simulink model "Rocket_Active_Airbrake_6DOF"  (R2026a)
settings: Solver=ode4  StopTime=28.0  FixedStep=0.002
PreLoadFcn:
  | init_airbrake_params
settings Model: Creator=wen-chungcheng  LastModifiedBy=wen-chungcheng

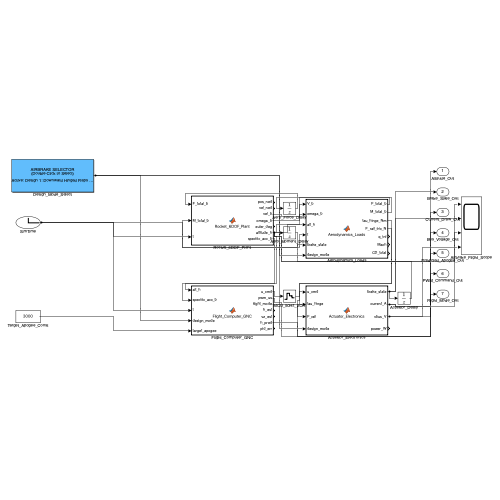
[thumbnail: Simulink's stored preview of the top-level diagram]
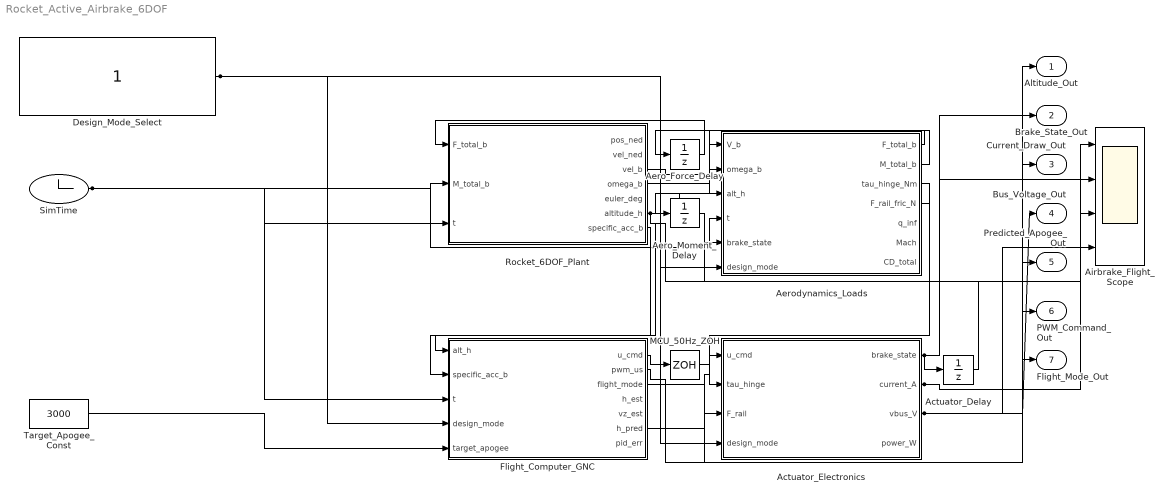
== system Rocket_Active_Airbrake_6DOF ==
  Actuator_Delay : UnitDelay  SampleTime=0.002
  Actuator_Electronics : MATLAB Function  TreatAsAtomicUnit=on
  Aero_Force_Delay : UnitDelay  InitialCondition=[0; 0; 0]  SampleTime=0.002
  Aero_Moment_Delay : UnitDelay  InitialCondition=[0; 0; 0]  SampleTime=0.002
  Aerodynamics_Loads : MATLAB Function  TreatAsAtomicUnit=on
  Airbrake_Flight_Scope : Scope  NumInputPorts=4
  Design_Mode_Select : Constant  mask(Airbrake Design Selector){design_popup=Design 1: Downward Hinged Flaps (0 - 90 deg, Savox SC-1258TG)}
      mask prompts: design_popup "Active Airbrake Mechanism:"
      mask help:
      | Choose active airbrake mechanism for 6-DOF simulation:
      | - Design 1: Downward Hinged Flaps (0 to 90 deg, Savox SC-1258TG)
      | - Design 2: Radially Outward Sliding Flaps (90 deg constant, Actuonix L16-R)
      mask init:
      | choice = get_param(gcb, 'design_popup');
      | if contains(choice, 'Design 1')
      |     val_internal = 1;
      | else
      |     val_internal = 2;
      | end
      settings: OpenFcn=open_system(gcb, 'mask');
      mask TypeOptions design_popup: Design 1: Downward Hinged Flaps (0 - 90 deg, Savox SC-1258TG) | Design 2: Radially Outward Sliding Flaps (90 deg, Actuonix L16-R)
      mask Display: disp(sprintf('AIRBRAKE SELECTOR\\n(Double-Click to Select)\\n\\nActive: %s', design_popup));
  Flight_Computer_GNC : MATLAB Function  TreatAsAtomicUnit=on
  MCU_50Hz_ZOH : ZeroOrderHold  SampleTime=0.02
  Rocket_6DOF_Plant : MATLAB Function  TreatAsAtomicUnit=on
  SimTime : Clock
  Target_Apogee_Const : Constant  Value=3000
  Altitude_Out : Outport
  Brake_State_Out : Outport  Port=2
  Current_Draw_Out : Outport  Port=3
  Bus_Voltage_Out : Outport  Port=4
  Predicted_Apogee_Out : Outport  Port=5
  PWM_Command_Out : Outport  Port=6
  Flight_Mode_Out : Outport  Port=7
  wires:
  SimTime/1 -> Rocket_6DOF_Plant/3(t), Aerodynamics_Loads/4(t), Flight_Computer_GNC/3(t)
  Design_Mode_Select/1 -> Aerodynamics_Loads/6(design_mode), Actuator_Electronics/4(design_mode), Flight_Computer_GNC/4(design_mode)
  Target_Apogee_Const/1 -> Flight_Computer_GNC/5(target_apogee)
  Aerodynamics_Loads/1(F_total_b) -> Aero_Force_Delay/1
  Aero_Force_Delay/1 -> Rocket_6DOF_Plant/1(F_total_b)
  Aerodynamics_Loads/2(M_total_b) -> Aero_Moment_Delay/1
  Aero_Moment_Delay/1 -> Rocket_6DOF_Plant/2(M_total_b)
  Rocket_6DOF_Plant/3(vel_b) -> Aerodynamics_Loads/1(V_b)
  Rocket_6DOF_Plant/4(omega_b) -> Aerodynamics_Loads/2(omega_b)
  Rocket_6DOF_Plant/6(altitude_h) -> Aerodynamics_Loads/3(alt_h), Flight_Computer_GNC/1(alt_h), Altitude_Out/1, Airbrake_Flight_Scope/1
  Rocket_6DOF_Plant/7(specific_acc_b) -> Flight_Computer_GNC/2(specific_acc_b)
  Aerodynamics_Loads/3(tau_hinge_Nm) -> Actuator_Electronics/2(tau_hinge)
  Aerodynamics_Loads/4(F_rail_fric_N) -> Actuator_Electronics/3(F_rail)
  Flight_Computer_GNC/1(u_cmd) -> MCU_50Hz_ZOH/1
  MCU_50Hz_ZOH/1 -> Actuator_Electronics/1(u_cmd)
  Actuator_Electronics/1(brake_state) -> Actuator_Delay/1, Brake_State_Out/1, Airbrake_Flight_Scope/2
  Actuator_Delay/1 -> Aerodynamics_Loads/5(brake_state)
  Actuator_Electronics/2(current_A) -> Current_Draw_Out/1, Airbrake_Flight_Scope/3
  Actuator_Electronics/3(vbus_V) -> Bus_Voltage_Out/1, Airbrake_Flight_Scope/4
  Flight_Computer_GNC/6(h_pred) -> Predicted_Apogee_Out/1
  Flight_Computer_GNC/2(pwm_us) -> PWM_Command_Out/1
  Flight_Computer_GNC/3(flight_mode) -> Flight_Mode_Out/1

== matlab function Rocket_Active_Airbrake_6DOF/Aerodynamics_Loads ==
  data: V_b input size=[3, 1]; F_total_b output size=[3, 1]; omega_b input size=[3, 1]; alt_h input size=1; t input size=1; brake_state input size=1; design_mode input size=1; M_total_b output size=[3, 1]; tau_hinge_Nm output size=1; F_rail_fric_N output size=1; q_inf output size=1; Mach output size=1; CD_total output size=1
function [F_total_b, M_total_b, tau_hinge_Nm, F_rail_fric_N, q_inf, Mach, CD_total] = Aerodynamics_Loads(V_b, omega_b, alt_h, t, brake_state, design_mode)
%#codegen
F_total_b = zeros(3,1);
M_total_b = zeros(3,1);
tau_hinge_Nm = 0.0;
F_rail_fric_N = 0.0;
q_inf = 0.0;
Mach = 0.0;
CD_total = 0.38;

h_m = max(0.0, min(20000.0, alt_h));
T_a = 288.15 - 0.0065 * h_m;
P_a = 101325.0 * ((max(0.1, 1.0 - (0.0065 * h_m) / 288.15))^5.2559);
rho = P_a / (287.05 * T_a);
a_s = sqrt(1.4 * 287.05 * T_a);
V_inf = max(0.1, norm(V_b));
Mach = V_inf / a_s;
q_inf = 0.5 * rho * (V_inf^2);
alpha = atan2(V_b(3), max(V_b(1), 0.1));
beta  = asin(max(-1.0, min(1.0, V_b(2) / V_inf)));
A_ref = 0.00817; D_body = 0.102; CD0 = 0.38; CNa = 5.80; Cmq = -26.0; Cnr = -26.0; Clp = -0.75;
x_CP = 1.88; x_CG_dry = 1.42;

% Clean drag rise
if Mach < 0.8
    CD_comp = CD0 / sqrt(max(0.1, 1 - Mach^2));
elseif Mach <= 1.1
    CD_comp = CD0 * (1.0 + 2.2 * ((Mach - 0.8)/0.3)^2);
else
    CD_comp = CD0 * (1.6 / sqrt(max(0.1, Mach^2 - 1)));
end

dCD_brakes = 0.0;
tau_hinge_Nm = 0.0;
F_rail_fric_N = 0.0;

if design_mode == 1
    % Design 1: Hinged flaps (0 - 90 deg)
    theta_rad = max(0.0, min(pi/2, brake_state));
    A_proj = 4.0 * (0.038 * 0.060) * sin(theta_rad);
    dCD_brakes = 1.25 * (sin(theta_rad)^2) * (A_proj / A_ref);
    F_flap = q_inf * 1.25 * sin(theta_rad) * (0.038 * 0.060);
    tau_hinge_Nm = (4.0 * F_flap * 0.028 * sin(theta_rad)) / 1.25;
else
    % Design 2: Sliding flaps at 90 deg (0 - 35 mm)
    s_m = max(0.0, min(0.035, brake_state));
    A_proj = 4.0 * 0.038 * s_m;
    dCD_brakes = 1.28 * (A_proj / A_ref);
    F_flap_norm = q_inf * 1.28 * (0.038 * s_m);
    F_rail_fric_N = 4.0 * (0.20 * F_flap_norm + 2.0);
end
CD_total = CD_comp + dCD_brakes;

% Thrust profile
t_lut = [0.0, 0.15, 0.40, 2.70, 3.05, 3.20];
T_lut = [0.0, 1680.0, 1380.0, 1260.0, 480.0, 0.0];
if t <= 3.20
    T_curr = interp1(t_lut, T_lut, t, 'linear', 0.0);
else
    T_curr = 0.0;
end

Fx_aero = -q_inf * A_ref * CD_total * cos(alpha) * cos(beta);
Fy_aero = -q_inf * A_ref * 5.80 * beta;
Fz_aero = -q_inf * A_ref * CNa * alpha;
F_total_b = [Fx_aero + T_curr; Fy_aero; Fz_aero];

SM = (x_CP - x_CG_dry) / D_body;
Mx_aero = q_inf * A_ref * D_body * (Clp * (omega_b(1) * D_body / (2 * V_inf)));
My_aero = q_inf * A_ref * D_body * (-CNa * SM * alpha + Cmq * (omega_b(2) * D_body / (2 * V_inf)));
Mz_aero = q_inf * A_ref * D_body * (+CNa * SM * beta + Cnr * (omega_b(3) * D_body / (2 * V_inf)));
M_total_b = [Mx_aero; My_aero; Mz_aero];

== matlab function Rocket_Active_Airbrake_6DOF/Rocket_6DOF_Plant ==
  data: F_total_b input size=[3, 1]; pos_ned output size=[3, 1]; M_total_b input size=[3, 1]; t input size=1; vel_ned output size=[3, 1]; vel_b output size=[3, 1]; omega_b output size=[3, 1]; euler_deg output size=[3, 1]; altitude_h output size=1; specific_acc_b output size=[3, 1]
function [pos_ned, vel_ned, vel_b, omega_b, euler_deg, altitude_h, specific_acc_b] = Rocket_6DOF_Plant(F_total_b, M_total_b, t)
%#codegen
% Explicit output preallocation
pos_ned = zeros(3,1);
vel_ned = zeros(3,1);
vel_b = zeros(3,1);
omega_b = zeros(3,1);
euler_deg = zeros(3,1);
altitude_h = 100.0;
specific_acc_b = zeros(3,1);

persistent r_ned V_b omega_b_st q on_rail dist_rail
if isempty(r_ned)
    r_ned = [0.0; 0.0; -100.0];
    V_b = [0.0; 0.0; 0.0];
    omega_b_st = [0.0; 0.0; 0.0];
    th0 = 86.0 * (pi/180);
    psi0 = 90.0 * (pi/180);
    q = [cos(th0/2)*cos(psi0/2); -sin(th0/2)*sin(psi0/2); sin(th0/2)*cos(psi0/2); cos(th0/2)*sin(psi0/2)];
    q = q / norm(q);
    on_rail = true;
    dist_rail = 0.0;
end
dt = 0.002;
m_dry = 8.20; m_prop_init = 1.95; t_burn = 3.20;
eta = min(1.0, max(0.0, t / t_burn));
m_curr = (m_dry + m_prop_init) - eta * m_prop_init;
I_wet = [0.022; 3.85; 3.85]; I_dry = [0.019; 2.95; 2.95];
I_diag = I_wet + eta * (I_dry - I_wet);
I_mat = diag(I_diag);

% DCM
q0=q(1); q1=q(2); q2=q(3); q3=q(4);
C_b_e = [ q0^2+q1^2-q2^2-q3^2, 2*(q1*q2+q0*q3), 2*(q1*q3-q0*q2);
          2*(q1*q2-q0*q3), q0^2-q1^2+q2^2-q3^2, 2*(q2*q3+q0*q1);
          2*(q1*q3+q0*q2), 2*(q2*q3-q0*q1), q0^2-q1^2-q2^2+q3^2 ];
C_e_b = C_b_e';
V_ned = C_e_b * V_b;
altitude_h = -r_ned(3);

if on_rail
    dist_rail = norm(r_ned - [0; 0; -100.0]);
    if dist_rail >= 3.65
        on_rail = false;
    end
end
F_eff_b = F_total_b;
M_eff_b = M_total_b;
if on_rail
    F_eff_b(2) = 0.0; F_eff_b(3) = 0.0;
    M_eff_b = [0; 0; 0];
    V_b(2) = 0.0; V_b(3) = 0.0;
    omega_b = [0; 0; 0];
end

% Gravity
F_grav_b = C_b_e * [0; 0; m_curr * 9.80665];
specific_acc_b = F_eff_b / m_curr;
F_sum_b = F_eff_b + F_grav_b;

% Derivatives
V_dot = (F_sum_b / m_curr) - cross(omega_b, V_b);
omega_dot = (M_eff_b - cross(omega_b, I_mat * omega_b)) ./ I_diag;
p=omega_b(1); q_r=omega_b(2); r=omega_b(3);
O_q = [0, -p, -q_r, -r; p, 0, r, -q_r; q_r, -r, 0, p; r, q_r, -p, 0];
q_dot = 0.5 * O_q * q;

% State updates
V_b = V_b + V_dot * dt;
omega_b = omega_b + omega_dot * dt;
q = q + q_dot * dt;
q = q / norm(q);
r_ned = r_ned + V_ned * dt;
pos_ned = r_ned;
vel_ned = V_ned;
vel_b = V_b;
omega_b = omega_b;
altitude_h = -r_ned(3);

% Euler angles
sin_p = max(-1.0, min(1.0, -2.0*(q(2)*q(4) - q(1)*q(3))));
pitch_deg = asin(sin_p) * 180/pi;
roll_deg  = atan2(2.0*(q(3)*q(4) + q(1)*q(2)), q(1)^2 - q(2)^2 - q(3)^2 + q(4)^2) * 180/pi;
yaw_deg   = atan2(2.0*(q(2)*q(3) + q(1)*q(4)), q(1)^2 + q(2)^2 - q(3)^2 - q(4)^2) * 180/pi;
euler_deg = [roll_deg; pitch_deg; yaw_deg];

== matlab function Rocket_Active_Airbrake_6DOF/Actuator_Electronics ==
  data: u_cmd input size=1; brake_state output size=1; tau_hinge input size=1; F_rail input size=1; design_mode input size=1; current_A output size=1; vbus_V output size=1; power_W output size=1
function [brake_state, current_A, vbus_V, power_W] = Actuator_Electronics(u_cmd, tau_hinge, F_rail, design_mode)
%#codegen
brake_state = 0.0;
current_A = 0.18;
vbus_V = 8.40;
power_W = 1.51;

persistent state
if isempty(state)
    state = [0.0; 0.0];
end
dt = 0.002;
cmd = max(0.0, min(1.0, u_cmd));
i_base = 0.18;

if design_mode == 1
    % Savox SC-1258TG Digital Titanium-Gear Servo
    th = state(1);
    th_dot = state(2);
    th_tgt = cmd * (pi/2);
    wn = 52.0; zeta = 0.72;
    th_ddot = (wn^2)*(th_tgt - th) - 2*zeta*wn*th_dot;
    w_max = 750 * (pi/180);
    pred_dot = th_dot + th_ddot * dt;
    if abs(pred_dot) > w_max
        pred_dot = sign(pred_dot) * w_max;
        th_ddot = (pred_dot - th_dot) / dt;
    end
    th = max(0.0, min(pi/2, th + th_dot*dt));
    th_dot = pred_dot;
    state = [th; th_dot];
    brake_state = th;
    i_act = 0.09 + 0.85 * (abs(th_dot)/w_max) + 2.75 * min(1.0, tau_hinge / 1.47);
else
    % Actuonix L16-R Micro Linear Actuator
    s = state(1);
    s_dot = state(2);
    s_tgt = cmd * 0.035;
    v_max = 0.032 * max(0.1, 1.0 - min(1.0, F_rail / 50.0));
    v_cmd = max(-v_max, min(v_max, (s_tgt - s)/0.03));
    s_ddot = (v_cmd - s_dot) / 0.03;
    s = max(0.0, min(0.035, s + s_dot*dt));
    s_dot = s_dot + s_ddot*dt;
    state = [s; s_dot];
    brake_state = s;
    i_act = 0.04 + 0.42 * (abs(s_dot)/0.032) + 0.68 * min(1.0, F_rail / 50.0);
end
current_A = i_base + i_act;
vbus_V = 8.40 - current_A * 0.045;
power_W = vbus_V * current_A;

== matlab function Rocket_Active_Airbrake_6DOF/Flight_Computer_GNC ==
  data: alt_h input size=1; u_cmd output size=1; specific_acc_b input size=[3, 1]; t input size=1; design_mode input size=1; target_apogee input size=1; pwm_us output size=1; flight_mode output size=1; h_est output size=1; vz_est output size=1; h_pred output size=1; pid_err output size=1
function [u_cmd, pwm_us, flight_mode, h_est, vz_est, h_pred, pid_err] = Flight_Computer_GNC(alt_h, specific_acc_b, t, design_mode, target_apogee)
%#codegen
u_cmd = 0.0;
pwm_us = 1000.0;
flight_mode = 0.0;
h_est = alt_h;
vz_est = 0.0;
h_pred = alt_h;
pid_err = 0.0;

persistent kf_x kf_P f_mode t_bo pid_I pid_prev_e pid_prev_d u_prev h_pred_filt
if isempty(kf_x)
    kf_x = [alt_h; 0.0];
    kf_P = [1.0, 0.0; 0.0, 4.0];
    f_mode = 0.0;
    t_bo = 0.0;
    pid_I = 0.0;
    pid_prev_e = 0.0;
    pid_prev_d = 0.0;
    u_prev = 0.0;
    h_pred_filt = alt_h;
end
dt = 0.002;
h_meas = alt_h;
ax_meas = specific_acc_b(1);

% 1D Kalman Filter
az_in = ax_meas - 9.80665;
A_k = [1.0, dt; 0.0, 1.0];
B_k = [0.5*dt^2; dt];
x_p = A_k * kf_x + B_k * az_in;
P_p = A_k * kf_P * A_k' + [0.25*dt^4, 0.5*dt^3; 0.5*dt^3, dt^2] * 2.5;
K = (P_p * [1; 0]) / (P_p(1,1) + 0.0144);
kf_x = x_p + K * (h_meas - x_p(1));
kf_P = (eye(2) - K * [1, 0]) * P_p;
h_est = kf_x(1);
vz_est = kf_x(2);

% State Machine
if f_mode == 0 && t > 0.05 && ax_meas > 15.0
    f_mode = 1.0;
end
if f_mode == 1 && ((t >= 2.8 && ax_meas < -5.0) || t >= 3.3)
    f_mode = 2.0;
    t_bo = t;
end
if f_mode == 2 && (t - t_bo) >= 0.30
    f_mode = 3.0;
end
if f_mode == 3 && (vz_est <= 15.0 || vz_est <= 1.0)
    f_mode = 4.0;
end

u_cmd = 0.0;
pid_err = 0.0;
h_pred = h_est;

if f_mode == 3
    h_m = max(0.0, min(20000.0, h_est));
    T_a = 288.15 - 0.0065 * h_m;
    P_a = 101325.0 * ((max(0.1, 1.0 - (0.0065 * h_m) / 288.15))^5.2559);
    rho = P_a / (287.05 * T_a);
    dh = (vz_est^2) / (2 * 9.80665);
    rho_eff = rho * exp(-0.5*dh / 8500.0);
    beta_clean = (rho_eff * 0.38 * 0.00817) / (2 * 8.2);
    h_pred_clean = h_est + (1.0 / (2*beta_clean)) * log(1.0 + (beta_clean/9.80665)*(vz_est^2));
    
    if design_mode == 1
        dCD = 1.25 * (sin(u_prev * pi/2)^3) * (0.00912 / 0.00817);
    else
        dCD = 1.28 * (0.00532 / 0.00817) * u_prev;
    end
    beta_curr = (rho_eff * (0.38 + dCD) * 0.00817) / (2 * 8.2);
    h_pred_raw = h_est + (1.0 / (2*beta_curr)) * log(1.0 + (beta_curr/9.80665)*(vz_est^2));
    
    h_pred_filt = 0.98 * h_pred_filt + 0.02 * h_pred_raw;
    h_pred = h_pred_filt;
    
    if h_pred_clean < target_apogee
        pid_err = h_pred_clean - target_apogee;
    else
        pid_err = h_pred - target_apogee;
    end
    
    P_term = 0.0035 * pid_err;
    d_err = (pid_err - pid_prev_e) / dt;
    D_term = (0.0008 * 25.0 * d_err + pid_prev_d) / (1.0 + 25.0 * dt);
    pid_prev_d = D_term;
    pid_prev_e = pid_err;
    
    tent_I = pid_I + 0.0012 * pid_err * dt;
    tent_u = P_term + tent_I + D_term;
    if tent_u >= 1.0
        if pid_err < 0, pid_I = tent_I; end
        u_pid = 1.0;
    elseif tent_u <= 0.0
        if pid_err > 0, pid_I = tent_I; end
        u_pid = 0.0;
    else
        pid_I = tent_I;
        u_pid = tent_u;
    end
    
    du = max(-3.0*dt, min(3.0*dt, u_pid - u_prev));
    u_cmd = max(0.0, min(1.0, u_prev + du));
    u_prev = u_cmd;
elseif f_mode == 4
    u_cmd = 0.0;
    u_prev = 0.0;
end

pwm_us = 1000.0 + u_cmd * 1000.0;
flight_mode = f_mode;
